simulink model "mpc_offsets"  (Simulink 7.0)
settings: Solver=ode23s  SolverMode=SingleTasking  StartTime=0.0  StopTime=Tstop  RelTol=1e-3
values from neighbouring files (symbols this model uses):
  r0 = 0    [mpc_switching_animation.m]    (also in mpcoffsets.m = 1.5*y0)
  x0 = zeros(4,1)    [afti16.m]    (also in mpc_pmmodel.m = xp0(:); mpc_switching_animation.m = x0([1 2]); mpccstr.m = [op_report.States(1).x;op_report.States(2).x]; mpcmotormodel.m)
libraries: mpclib x1
settings Model: Creator=jowen  LastModifiedBy=rchen  ExtModeTrigMode=oneshot  ExtModeArmWhenConnect=off
settings DataIOCC: LimitDataPoints=off  SignalLoggingName=sigsOut
settings OptimizationCC: BooleanDataType=off  InlineInvariantSignals=on
settings DebuggingCC: CheckExecutionContextPreStartOutputMsg=on  CheckExecutionContextRuntimeOutputMsg=on  SignalResolutionControl=TryResolveAllWithWarning  SolverPrmCheckMsg=none  MultiTaskDSMMsg=warning  MultiTaskCondExecSysMsg=none  IntegerOverflowMsg=none  StrictBusMsg=None
settings HardwareCC: TargetUnknown=on
settings RTWCC: IncludeERTFirstTime=on

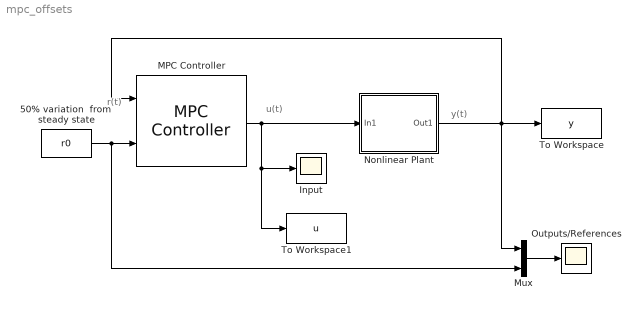
== system mpc_offsets ==
  note: u(t)
  note: y(t)
  note: r(t)
  50% variation  from  steady state : Constant  Value=r0  OutDataType=sfix(16)  OutScaling=2^0
  Input : Scope
      settings: TimeRange=10  YMin=-8  YMax=2  DataFormat=Structure
  MPC Controller : mpclib/MPC Controller  SystemSampleTime=-1  mpcobj=mpc_controller  n_mv=0  x0=[]  ref_from_ws=off  ref_signal_name=[]  ref_preview=on  md_from_ws=off  md_signal_name=[]  md_preview=on  from_project=off  md_inport=off  mv_inport=off  lims_inport=off  project_file=MPCtask.mat
  Mux : Mux  Inputs=2
  Nonlinear Plant : Subsystem
  Outputs/References : Scope
      settings: TimeRange=10  YMin=-0.8  YMax=-0.4  DataFormat=Structure
  To Workspace : ToWorkspace  VariableName=y  SampleTime=-1  SaveFormat=Structure With Time
      settings: MaxDataPoints=Inf
  To Workspace1 : ToWorkspace  VariableName=u  SampleTime=-1  SaveFormat=Structure With Time
      settings: MaxDataPoints=Inf
  wires:
  MPC Controller/1 -> Input/1, To Workspace1/1, Nonlinear Plant/1(In1)
  Mux/1 -> Outputs/References/1
  50% variation  from  steady state/1 -> Mux/2, MPC Controller/2
  Nonlinear Plant/1(Out1) -> To Workspace/1, Mux/1, MPC Controller/1

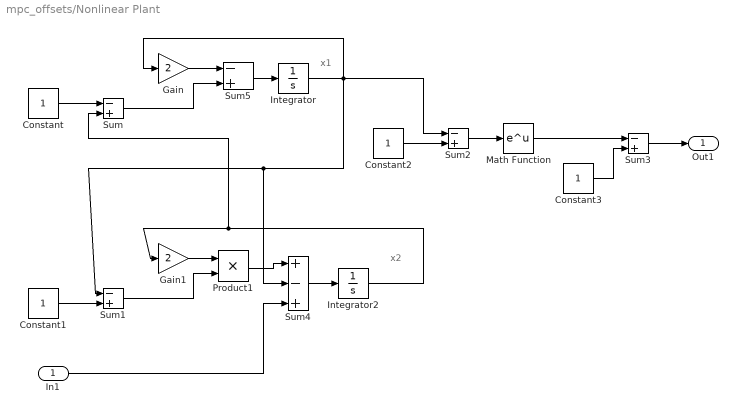
== system mpc_offsets/Nonlinear Plant ==
  note: x1
  note: x2
  In1 : Inport  OutDataType=sfix(16)  OutScaling=2^0
  Constant{,1..3} (4 alike) : Constant  OutDataType=sfix(16)  OutScaling=2^0
  Gain : Gain  Gain=2  ParameterDataType=sfix(16)  ParameterScaling=2^0  OutDataType=sfix(16)  OutScaling=2^0  SaturateOnIntegerOverflow=on
  Gain1 : Gain  Gain=2  ParameterDataType=sfix(16)  ParameterScaling=2^0  OutDataType=sfix(16)  OutScaling=2^0  SaturateOnIntegerOverflow=on
  Integrator : Integrator  InitialCondition=x0(1)  UpperSaturationLimit=Inf  LowerSaturationLimit=-Inf
  Integrator2 : Integrator  InitialCondition=x0(2)  UpperSaturationLimit=Inf  LowerSaturationLimit=-Inf
  Math Function : Math  OutDataType=sfix(16)  OutScaling=2^0  SaturateOnIntegerOverflow=on
  Product1 : Product  OutDataType=sfix(16)  OutScaling=2^0  SaturateOnIntegerOverflow=on  InputSameDT=on
  Sum{,1..3,5} (5 alike) : Sum  Inputs=-+  OutDataType=sfix(16)  OutScaling=2^0  SaturateOnIntegerOverflow=on  InputSameDT=on
  Sum4 : Sum  Inputs=+-+  OutDataType=sfix(16)  OutScaling=2^0  SaturateOnIntegerOverflow=on  InputSameDT=on
  Out1 : Outport  OutDataType=sfix(16)  OutScaling=2^0
  wires:
  Sum5/1 -> Integrator/1
  Gain/1 -> Sum5/1
  Integrator/1 -> Gain/1, Sum2/1, Sum1/1, Sum4/2
  Constant/1 -> Sum/1
  Sum/1 -> Sum5/2
  Gain1/1 -> Product1/1
  Sum1/1 -> Product1/2
  Constant1/1 -> Sum1/2
  Constant2/1 -> Sum2/2
  Sum2/1 -> Math Function/1
  Constant3/1 -> Sum3/2
  Math Function/1 -> Sum3/1
  Sum3/1 -> Out1/1
  Integrator2/1 -> Gain1/1, Sum/2
  Sum4/1 -> Integrator2/1
  Product1/1 -> Sum4/1
  In1/1 -> Sum4/3
